simulink model "ZController"  (R2017a)
settings: Solver=VariableStepAuto  StartTime=0.0  StopTime=10.0  RelTol=1e-3
settings Model: Creator=erich  LastModifiedBy=erich

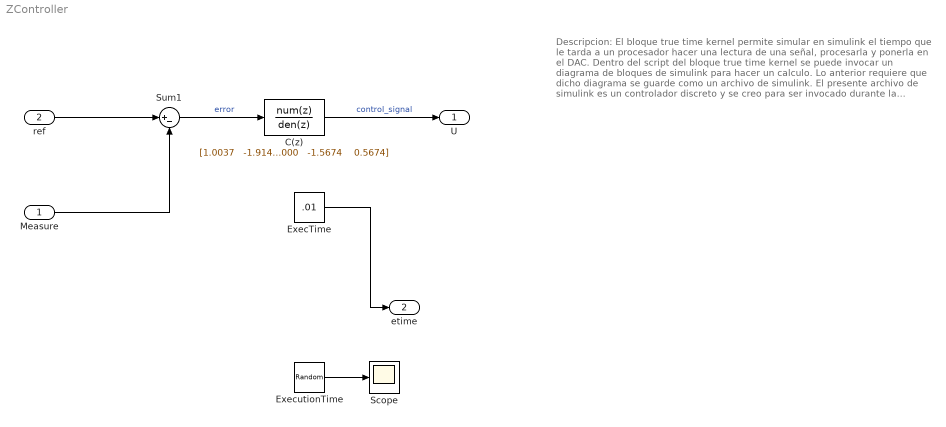
== system ZController ==
  note: Descripcion:
      | El bloque true time kernel permite simular
      | en simulink el tiempo que le tarda a un
      | procesador hacer una lectura de una señal,
      | procesarla y ponerla en el DAC. Dentro del
      | script del bloque true time kernel
      | se puede invocar un diagrama de bloques de
      | simulink para hacer un calculo. Lo anterior requiere
      | que dicho diagrama se guarde como un archivo de
      | simulink.
      |
      | El presente archivo de simulink es un
      | controlador discreto y se creo para ser invocado
      | durante la simulacion de blk_learn por el bloque
      | true time kernel.
      |
      | Execution time corresponde al tiempo que le toma
      | al procesador hacer el calculo del algoritmo de control.
      | En este caso se puso como variable aleatoria para
      | modelar que se trata de un procesador con multiples
      | tareas que pueden variar en el tiempo.
      |
      | Cuando la dispersion del numero aleatorio crece
      | por encima de .01 el desempeño del controlador se
      | degrada.
  Measure : Inport
  ref : Inport  Port=2
  C(z) : DiscreteTransferFcn  Numerator="[1.0037   -1.9141    0.9410]"  Denominator="[1.0000   -1.5674    0.5674]"  SampleTime=1
  ExecTime : Constant  Value=.01  SampleTime=1
  ExecutionTime : RandomNumber  Mean=.01  Variance=.02  Seed=.01  SampleTime=1
  Scope : Scope
  Sum1 : Sum  Inputs=|+-
  U : Outport
  etime : Outport  Port=2
  wires:
  Measure/1 -> Sum1/2
  ref/1 -> Sum1/1
  Sum1/1 -> C(z)/1  "error"
  C(z)/1 -> U/1  "control_signal"
  ExecTime/1 -> etime/1
  ExecutionTime/1 -> Scope/1
